simulink model "model5_cm"  (R2018b)
settings: Solver=FixedStepDiscrete  StartTime=0.0  StopTime=Inf  FixedStep=0.025  RelTol=1e-3  EnableMultiTasking=on
undefined symbols (not defined in the file): acA2000, Ace, Basler, FreeRun, PoCL, USETHISONE
libraries: dotFinder_ul x1, xpcbitflowlib x1, slrtlib x1, videoStream_ul x1, imageUDPNode_ul x1
settings Model: sg_rtwmakecfg_data=_bitflow_  SimulationMode=external  Creator=mcobb  LastModifiedBy=mae-ncsucore
settings SolverCC: ConcurrentTasks=on  AutoInsertRateTranBlk=on
settings DataIOCC: SaveFormat=StructureWithTime
settings OptimizationCC: BlockReduction=off  OptimizeBlockIOStorage=off  BufferReuse=off  GlobalBufferReuse=off  ExpressionFolding=off  LocalBlockOutputs=off  OptimizeDataStoreBuffers=off  BusAssignmentInplaceUpdate=off
settings DebuggingCC: LibraryContextMissingDiagnostic=none
settings HardwareCC: ProdBitPerPointer=32  ProdBitPerSizeT=32  ProdBitPerPtrDiffT=32  ProdLargestAtomicFloat=None  ProdWordSize=32  ProdLongLongMode=on  ProdHWDeviceType=Generic->32-bit x86 compatible
settings SFSimCC: SimUseLocalCustomCode=off
settings RTWCC: SystemTargetFile=slrt.tlc  TemplateMakefile=slrt_default_tmf  Description=Simulink Real-Time  RTWUseLocalCustomCode=off  CodeExecutionProfiling=on  RTWCompilerOptimization=on
settings SimulinkRealTimeCC: SupportVariableSizeSignals=on  PreserveStateflowLocalDataDimensions=off  RL32LogTETModifier=off  RL32ObjectName=tg5  xPCisDefaultEnv=off  xPCTargetPCEnvName=Machine5  xPCConcurrentTasks=on

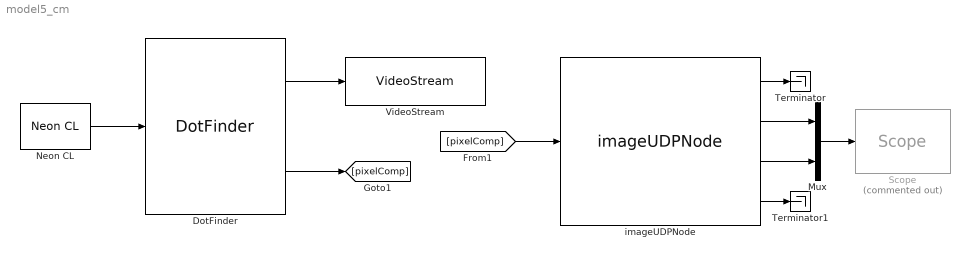
== system model5_cm ==
  DotFinder : dotFinder_ul/DotFinder  ROIPositionHoldEnable=off  ROIPositionHoldCoordinates=[300 800]  ROIDimVec_px=params.roiSlntSize_px.Value  ROIHalfDimVec_px=[25 50]  ROISplitDims_px=[1 50 ; 1 50 ; 1 50 ; 51 49]  DotOrientation=Horizontal  OverlayOutput=on  ImageDimensions=params.slntImageSize_px.Value  CrosshairPixelWidth_px=params.slntCrsHrWdth_px.Value
  Mux : Mux  Inputs=2
  "Neon CL " : xpcbitflowlib/Neon CL   camerapath=Basler-Ace-acA2000-340km-E2-PoCL-FreeRun-USETHISONE.r64  r64=CAMERA  sampletime=0.025  slot=-1  make=Basler  model=acA2000-340km  mode=8 bit, 2 tap, 2048x1088, Free Run  owner=BitFlow  revision=1  modelcomp=0  revcomp=0  aqtimeout=4096  format=1  flashmux=Mux_2TOEP  flashdcc=DCC  pixbitdepth=8  xsize=2048  ysize=1088  xstart=0  ystart=0  dx=2048  dy=1088  expmod="[1  0]"  config="[4294967295         128;4294967295           0;4294967295           0;4294967295           0;4294967295           0;4294967295           0;4294967295      262144;4294967295           0;4294967295           0;4294967295           0;4294967295        1024;4294967295           0;4294967295           0;4294967295  4294967295;4294967295           0;4294967295           0;4294967295           0;4294967295      737280;4294967295        1088;4294967295           0;4294967295           0;4294967295           0;4294967295           0;4294967295           0;4294967295           0;4294967295           0;4294967295        7372;4294967295           0]"  ctab="[4      0     16      1   4112      2     16  32768      0]"  qtabmodel="[1   2048  65536]"  trigmode=0  baud=1  bytewidth=4  parity=1  stopbits=1  command="\"\""  response=0  comments=|
      | Free Run Mode / CC Trigger Mode
      | 
      | CC Trigger can be adjusted via GPV0 in CTAB
      | 
      | To use CC Trigger, camera must set to CC Trigger Mode.
      settings: SourceProductName=Simulink Real-Time: Speedgoat I/O Driver Library
  "Scope " : slrtlib/Displays and Logging/Scope   Commented=on  scopeno=2  scopetype=Target  autostart=on  viewmode=Numerical  formatstr='%15.6f'  grid=on  ylimits=[0,0]  nosamples=250  noprepostsamples=0  interleave=1  triggermode=FreeRun  triggersignal=1  trigsignalfromport=off  triggerlevel=0.0  triggerslope=Either  triggerscope=1  triggersample=0  filename=data.dat  mode=Lazy  writesize=512  autorestart=off  dynamicfilemode=off  maxwritefilesize=512*1024^2
  Terminator : Terminator
  Terminator1 : Terminator
  VideoStream : videoStream_ul/VideoStream  enbl=on  decimationFactor=params.slntVidStrmDec_na.Value  resizeFactor=params.slntVidStrmImgWdth_px.Value
  imageUDPNode : imageUDPNode_ul/imageUDPNode  sample_time=0.025  IpAddress=30.30.30.3  toPort=params.slantToPort_na.Value  offset_threshold=params.offsetThreshold_s.Value  sync_interval=params.syncInterval_s.Value  min_pdelay_req_interval=params.slantMinDelay_s.Value  MaskUnpackedDataTypes={['double']}
  wires:
  DotFinder/2 -> [pixelComp]
  imageUDPNode/3 -> Mux/2
  imageUDPNode/2 -> Mux/1
  Mux/1 -> "Scope "/1
  DotFinder/1 -> VideoStream/1
  "Neon CL "/1 -> DotFinder/1
  [pixelComp] -> imageUDPNode/1
  imageUDPNode/1 -> Terminator/1
  imageUDPNode/4 -> Terminator1/1
